simulink model "traj_gen_sim"  (R2023a)
settings: Solver=FixedStepDiscrete  StartTime=0.0  StopTime=100  FixedStep=Ts  RelTol=1e-3
values from neighbouring files (symbols this model uses):
  T = out.tout    [fig_cartesian.m]
undefined symbols (not defined in the file or in its folder): DiscIntNeverNeededParam, P
libraries: simulink x2, robotcorelib x1, robotmaniplib x1, shareduavrstlib x1
settings Model: Creator=stt  LastModifiedBy=stt
settings OptimizationCC: ReuseModelBlockBuffer=off
settings ModelReferenceCC: EnableRefExpFcnMdlSchedulingChecks=on

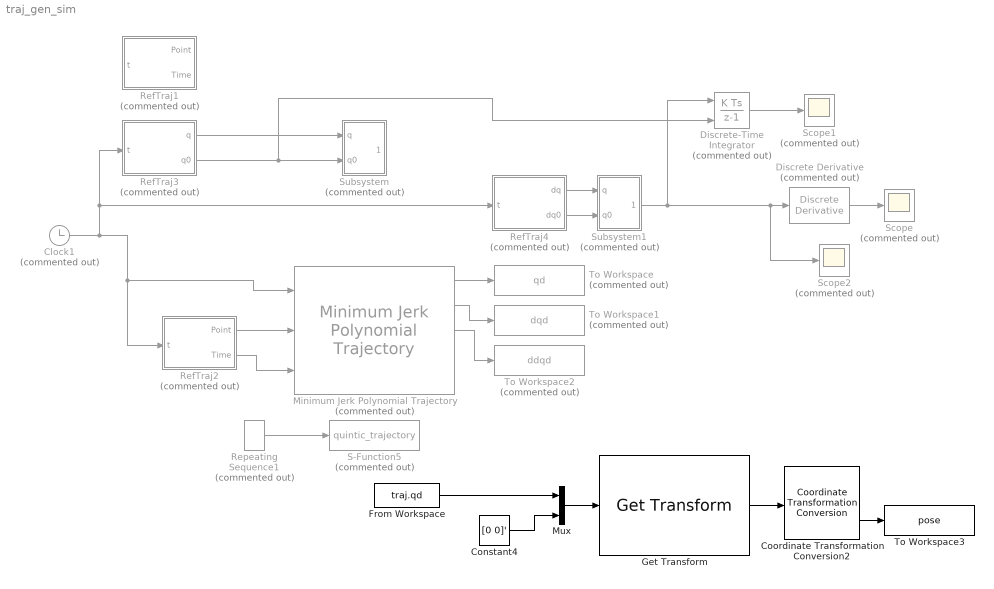
== system traj_gen_sim ==
  Clock1 : Clock  Commented=on
  Constant4 : Constant  Value=[0 0]'
  Coordinate Transformation Conversion2 : robotcorelib/Coordinate Transformation Conversion  InputRepresentation=Homogeneous Transformation  InputEulerSequence=ZYX  ShowTrVecInputPort=on  OutputRepresentation=Rotation Matrix  OutputEulerSequence=XYZ  ShowTrVecOutputPort=on  SimulateUsing=Interpreted execution
  Discrete Derivative : simulink/Discrete/Discrete Derivative  Commented=on  gainval=1.0  ICPrevScaledInput=0.0  OutMin=[]  OutMax=[]  OutDataType=fixdt(1, 16)  OutScaling=2^-10  DoSatur=off
  Discrete-Time Integrator : DiscreteIntegrator  Commented=on  InitialConditionSource=external  SampleTime=-1  ICPrevOutput=DiscIntNeverNeededParam  ICPrevScaledInput=DiscIntNeverNeededParam
  From Workspace : FromWorkspace  VariableName=traj.qd
  Get Transform : robotmaniplib/Get Transform  RigidBodyTree=panda  SourceBody=panda_link8  TargetBody=panda_link0  SimulateUsing=Interpreted execution
  Minimum Jerk Polynomial Trajectory : shareduavrstlib/Minimum Jerk Polynomial Trajectory  Commented=on  ShowBCInputPort=off  ShowPolynomialCoefs=off  ShowStatusOutputPort=off  TimeAllocation=off  TimeWeight=100  MinSegmentTime=0.1  MaxSegmentTime=1  MaxIteration=1500  MaxTime=10  SimulateUsing=Interpreted execution
  Mux : Mux  Inputs=2
  RefTraj1 : MATLAB Function  Commented=on  TreatAsAtomicUnit=on
  RefTraj2 : MATLAB Function  Commented=on  TreatAsAtomicUnit=on
  RefTraj3 : MATLAB Function  Commented=on  TreatAsAtomicUnit=on
  RefTraj4 : MATLAB Function  Commented=on  TreatAsAtomicUnit=on
  Repeating Sequence1 : simulink/Sources/Repeating Sequence  Commented=on  rep_seq_t=[0 105]  rep_seq_y=[0 105]
  S-Function5 : S-Function  Commented=on  FunctionName=quintic_trajectory  Parameters=P,T  SFunctionDeploymentMode=off  EnableBusSupport=off
  Scope : Scope  Commented=on
  Scope1 : Scope  Commented=on
  Scope2 : Scope  Commented=on
  Subsystem : Subsystem  Commented=on
  Subsystem1 : Subsystem  Commented=on
  To Workspace : ToWorkspace  Commented=on  VariableName=qd  SaveFormat=Timeseries  SampleTime=-1
  To Workspace1 : ToWorkspace  Commented=on  VariableName=dqd  SaveFormat=Timeseries  SampleTime=-1
  To Workspace2 : ToWorkspace  Commented=on  VariableName=ddqd  SaveFormat=Timeseries  SampleTime=-1
  To Workspace3 : ToWorkspace  VariableName=pose  SaveFormat=Timeseries  SampleTime=-1
  wires:
  Get Transform/1 -> Coordinate Transformation Conversion2/1
  Coordinate Transformation Conversion2/2 -> To Workspace3/1
  Constant4/1 -> Mux/2
  Mux/1 -> Get Transform/1
  From Workspace/1 -> Mux/1
  Repeating Sequence1/1 -> S-Function5/1
  RefTraj2/1(Point) -> Minimum Jerk Polynomial Trajectory/2
  RefTraj2/2(Time) -> Minimum Jerk Polynomial Trajectory/3
  Clock1/1 -> RefTraj4/1(t), RefTraj3/1(t), RefTraj2/1(t), Minimum Jerk Polynomial Trajectory/1
  RefTraj3/1(q) -> Subsystem/1(q)
  RefTraj3/2(q0) -> Discrete-Time Integrator/2, Subsystem/2(q0)
  RefTraj4/2(dq0) -> Subsystem1/2(q0)
  RefTraj4/1(dq) -> Subsystem1/1(q)
  Subsystem1/1(Out1) -> Discrete-Time Integrator/1, Scope2/1, Discrete Derivative/1
  Discrete Derivative/1 -> Scope/1
  Discrete-Time Integrator/1 -> Scope1/1
  Minimum Jerk Polynomial Trajectory/1 -> To Workspace/1
  Minimum Jerk Polynomial Trajectory/2 -> To Workspace1/1
  Minimum Jerk Polynomial Trajectory/3 -> To Workspace2/1

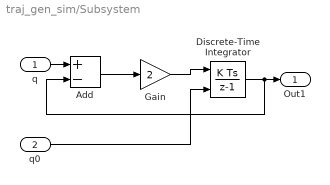
== system traj_gen_sim/Subsystem ==
  q : Inport
  q0 : Inport  Port=2
  Add : Sum  Inputs=+-
  Discrete-Time Integrator : DiscreteIntegrator  InitialConditionSource=external  SampleTime=-1  ICPrevOutput=DiscIntNeverNeededParam  ICPrevScaledInput=DiscIntNeverNeededParam
  Gain : Gain  Gain=2
  Out1 : Outport
  wires:
  Gain/1 -> Discrete-Time Integrator/1
  Add/1 -> Gain/1
  Discrete-Time Integrator/1 -> Out1/1, Add/2
  q/1 -> Add/1
  q0/1 -> Discrete-Time Integrator/2

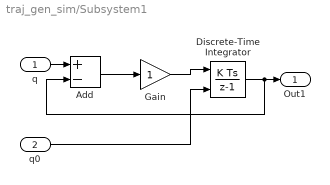
== system traj_gen_sim/Subsystem1 ==
  q : Inport
  q0 : Inport  Port=2
  Add : Sum  Inputs=+-
  Discrete-Time Integrator : DiscreteIntegrator  InitialConditionSource=external  SampleTime=-1  ICPrevOutput=DiscIntNeverNeededParam  ICPrevScaledInput=DiscIntNeverNeededParam
  Gain : Gain
  Out1 : Outport
  wires:
  Gain/1 -> Discrete-Time Integrator/1
  Add/1 -> Gain/1
  Discrete-Time Integrator/1 -> Out1/1, Add/2
  q/1 -> Add/1
  q0/1 -> Discrete-Time Integrator/2

== matlab function traj_gen_sim/RefTraj2 ==
  data: Point output; Time output; t input
function [Point,Time] = fcn(t)

q0=[0.0,  -0.6, -0.00,-2.25, 0.00, 1.5, 0.80]';
q1=[-0.75, 0.25, 0,   -1.3, -1.2,  0.85,-1.3]';
q2=[1.5,   0.6, -0.83,-0.8,  1.04, 1.6,-1.0]';
q3=[0.25, -0.55, 0.3, -1.75, 0.25, 1.25,0.5]';
q4=[-1.2, -0.84,-0.85,-1.0,  1.07, 2.55,1.05]';
q5=[-2.25,-1.2,  2.23,-0.63,-0.54, 2.07, 1.50]';
q6=[-0.25,-0.56,-0.23,-1.33,-0.24, 2.0, 0.5]';
q7=[0.25,-0.55,0.3,-1.75,1.25,0.75,0.5]';
q8=[-0.75,0.25,0,-0.8,-1.2,0.5,-1.8]';
q9=[-0.25,1.0,-0.23,-1.33,-1.24,1.1,-1.8]';

% q0 = [0.0,-0.6,-0.00,-2.25,0.00,1.5,0.80]';
% q1=[0.25,-0.55,0.3,-1.75,1.25,0.75,0.5]';
% q2=[1.5,0.6,-0.83,-1.5,1.04,1.6,-1.75]';
% q3=[-0.75,0.25,0,-0.8,-1.2,0.5,-1.8]';
% q4=[-1.2,-0.84,-0.85,-1.0,1.07,2.55,2.05]';
% q5=[-2.25,-1.2,2.23,-0.73,-1.54,2.8,1.50]';
% q6=[-0.25,1.0,-0.23,-1.33,-1.24,1.1,-1.8]';


q = [q0,q1,q2,q3,q4,q5,q6,q7,q8,q9,q0,...
   q0,q9,q7,q8,q6,q4,q5,q3,q1,q2,q0];
% q=[q0,q1,q2,q3,q4,q5,q6,q0,...
%     q0,q2,q4,q6,q1,q3,q5,q0];
%T = [0,4,8,12,16,20,25,30,80,83,86,89,92,95,98,100];
T1=[0,3,6,8,12,15,18,21,24,27,30];
T2=T1+70;%[70,74,78,81,85,90,95,100];

if t<30
    Point=q(:,1:11);
    Time=T1(1:11);
elseif t>T2(1) && t<=T2(end)
    Point=q(:,12:22);
    Time=T2(1:11);
else
    Point=q0*ones(1,11);
    Time=linspace(T1(end),T2(1),11);
end

== matlab function traj_gen_sim/RefTraj3 ==
  data: q output; t input; q0 output
function [q,q0] = fcn(t)

q0=[0.0,  -0.6, -0.00,-2.25, 0.00, 1.5, 0.80]';
% q1=[0.2, -0.8, -0.3,   -2.05, 0.2,  1.3,0.6]';
% q2=[0.4, -1, -0.5,   -1.9,  0.5, 1.2, 0.4]';
% q3=[0.6, -1.2, 0.8, -1.7, 0.7, 1.05,0.2]';
if t<=5
    q=q0;
elseif t<=25
    q=0.05*tanh(t-15)+q0;
elseif t<=30
    q=q0+1;
elseif t<=50
    q=-0.05*tanh(t-40)+q0+1;
else
    q=q0;
end

== matlab function traj_gen_sim/RefTraj4 ==
  data: dq output; t input; dq0 output
function [dq,dq0] = fcn(t)

dq0=zeros(7,1);v=0.1;
% q1=[0.2, -0.8, -0.3,   -2.05, 0.2,  1.3,0.6]';
% q2=[0.4, -1, -0.5,   -1.9,  0.5, 1.2, 0.4]';
% q3=[0.6, -1.2, 0.8, -1.7, 0.7, 1.05,0.2]';
if t<=9
    dq=dq0;
elseif t<=10
    dq=v*tanh(t-9)/tanh(1)*ones(7,1)+dq0;
elseif t<20
    dq=v*ones(7,1);
elseif t<21
    dq=-v*tanh(t-20)/tanh(1)*ones(7,1)+v*ones(7,1);
elseif t<29
    dq=dq0;
elseif t<30
    dq=-v*tanh(t-29)/tanh(1)*ones(7,1)+dq0;
elseif t<40
    dq=-v*ones(7,1);
elseif t<41
    dq=v*tanh(t-40)/tanh(1)*ones(7,1)-v*ones(7,1);
else
    dq=dq0;


end

== matlab function traj_gen_sim/RefTraj1 ==
  data: Point output; Time output; t input
function [Point,Time] = fcn(t)

q0=[0.0,  -0.6, -0.00,-2.25, 0.00, 1.5, 0.80]';
% q1=[0.2, -0.8, -0.3,   -2.05, 0.2,  1.3,0.6]';
% q2=[0.4, -1, -0.5,   -1.9,  0.5, 1.2, 0.4]';
% q3=[0.6, -1.2, 0.8, -1.7, 0.7, 1.05,0.2]';

if t<10
    


q = [q0,q1,q2,q3,q2,q1,q0];
T = [0,3,6,9,12,15,18,...
    20,23,26,29,32,35,38,...
    40,43,46,49,52,55,58];

if t<20
    Point=q;
    Time=T(1:7);
elseif t<40 
    Point=q;
    Time=T(8:14);
else
    Point=q;
    Time=T(15:21);
end
